simulink model "Utkarsh_2005574_W1_P6_Ref_Model"  (R2020b)
settings: Solver=FixedStepDiscrete  StartTime=0.0  StopTime=10.0  FixedStep=0.2  RelTol=1e-3
settings Model: Creator=home  LastModifiedBy=home
settings DataIOCC: ExternalInput=[t,u]  SaveOutput=off  SaveTime=off

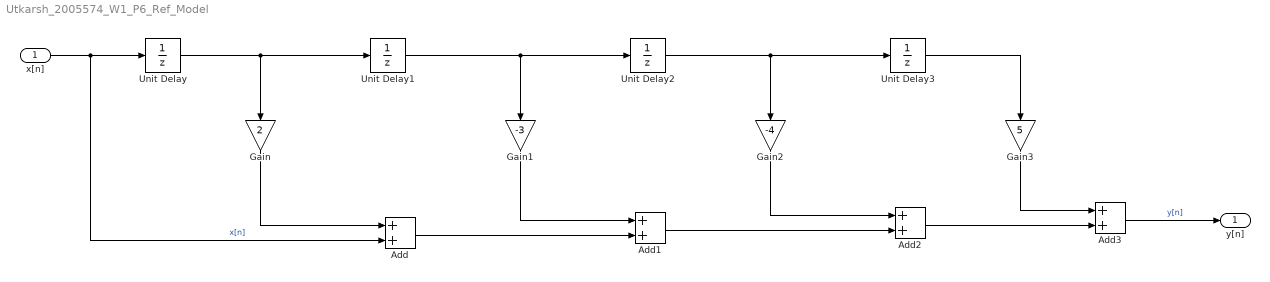
== system Utkarsh_2005574_W1_P6_Ref_Model ==
  x[n] : Inport  OutDataTypeStr=double  PortDimensions=1  SampleTime=[0.20000000000000001,0]
  Add{,1..3} (4 alike) : Sum
  Gain : Gain  Gain=2
  Gain1 : Gain  Gain=-3
  Gain2 : Gain  Gain=-4
  Gain3 : Gain  Gain=5
  Unit Delay{,1..3} (4 alike) : UnitDelay  SampleTime=-1  HasFrameUpgradeWarning=on
  y[n] : Outport  OutDataTypeStr=double  PortDimensions=1  SampleTime=[0.20000000000000001,0]
  wires:
  Gain2/1 -> Add2/1
  Unit Delay1/1 -> Gain1/1, Unit Delay2/1
  Gain/1 -> Add/1
  Unit Delay/1 -> Gain/1, Unit Delay1/1
  x[n]/1 -> Add/2, Unit Delay/1  "x[n]"
  Gain1/1 -> Add1/1
  Add/1 -> Add1/2
  Add1/1 -> Add2/2
  Unit Delay3/1 -> Gain3/1
  Add2/1 -> Add3/2
  Gain3/1 -> Add3/1
  Unit Delay2/1 -> Unit Delay3/1, Gain2/1
  Add3/1 -> y[n]/1  "y[n]"
